simulink model "ssc_pneumatic_actuator"  (R2014a)
settings: Solver=ode23t  StartTime=0.0  StopTime=10  FixedStep=0.01  RelTol=1e-3
undefined symbols (not defined in the file): sigbuilder_block
libraries: fl_lib x50, nesl_utility x8
Description:
  | Pneumatic Actuation Circuit
  | 
  | This example shows how the Foundation Library pneumatic components
  | can be used to model a controlled pneumatic actuator. The Directional
  | 5-way valve, Double-acting pneumatic actuator and Pipe blocks
  | are masked subsystems created from Foundation Library blocks.
  | Double-click on the blocks to view the subsystem parameters. Select
  | the block and type ctrl-U to view its construction from fundamental
  | components. The pipe and actuator components include a simple
  | convection model of heat loss.
  | 
  | In the simulation, the directional valve is initially moved to its
  | maximum positive displacement, and the actuator moves the load
  | until it reaches the actuator end stop. The valve is then centered, and
  | the load is held. Next the valve moves to its maximum negative
  | displacement and the actuator retracts to its minimum length. The
  | valve is then centered again, locking the load in position.
  | 
  | 
  | Copyright 2008-2014 The MathWorks, Inc.
settings Model: Creator=MathWorks  LastModifiedBy=rodralez
settings DataIOCC: SignalLoggingSaveFormat=ModelDataLogs
settings OptimizationCC: ExpressionDepthLimit=2147483647
settings DebuggingCC: UnderspecifiedInitializationDetection=Classic  SolverPrmCheckMsg=none  FcnCallInpInsideContextMsg=UseLocalSettings  StateNameClashWarn=warning  StrictBusMsg=Warning
settings GRTTargetCC: CombineOutputUpdateFcns=off  GRTInterface=on

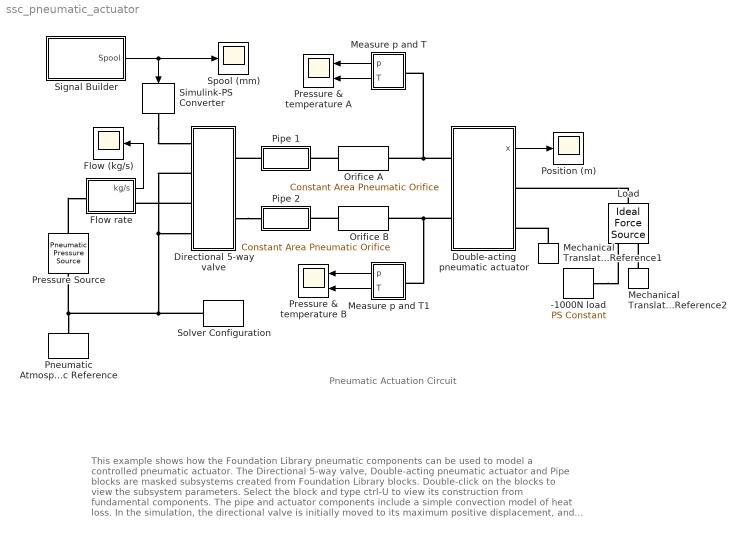
== system ssc_pneumatic_actuator ==
  note: Pneumatic Actuation Circuit
  note: This example shows how the Foundation Library pneumatic components can be used to model a controlled
      | pneumatic actuator. The Directional 5-way valve, Double-acting pneumatic actuator and Pipe blocks
      | are masked subsystems created from Foundation Library blocks. Double-click on the blocks to view
      | the subsystem parameters. Select the block and type ctrl-U to view its construction from fundamental
      | components. The pipe and actuator components include a simple convection model of heat loss.
      | In the simulation, the directional valve is initially moved to its maximum positive displacement,
      | and the actuator moves the load until it reaches the actuator end stop. The valve is then centered,
      | and the load is held. Next the valve moves to its maximum negative displacement and the actuator
      | retracts to its minimum length. The valve is then centered again, locking the load in position.
  -1000N load : fl_lib/Physical Signals/Sources/PS Constant  constant=-1000
  Directional 5-way valve : Subsystem  mask(Directional 5-way valve){Cd=0.82, x_max=5, A_max=5, x_lap=0.2, A_leak=0.0001}
      mask prompts: Cd "Discharge coefficient:"; x_max "Displacement limit (mm)"; A_max "Maximum orifice area (mm^2)"; x_lap "Displacement range for leakage (mm)"; A_leak "Leakage area at x=0 (mm^2)"
      mask help: Models a directional 5-way valve assuming a linear relationship between valve position and valve area. Input supply pressure should be applied to port P, and the actuator connected to ports A and B. Ports R and S are the return paths for ports A and B respectively.
      mask Display:
      | image(imread('valve_5_3.jpg'))
      | color('red')
      | port_label('Lconn',1,'x')
      | port_label('Lconn',2,'R')
      | port_label('Lconn',3,'P')
      | port_label('Lconn',4,'S')
      | port_label('Rconn',1,'A')
      | port_label('Rconn',2,'B')
  Double-acting pneumatic actuator : Subsystem  mask(Double-acting pneumatic actuator){A=0.002, L=0.2, V0=1e-4, mass=1, lambda=200, mass_total=3, c_act=870, k=100, Ta=293.15, x0=0, p0_A=101325, T_A=293.15, p0_B=101325, T_B=293.15, T_act=293.15}
      mask prompts: A "Cross-sectional area (m^2)"; L "Length of travel (m)"; V0 "Dead volume (m^3)"; mass "Piston mass (kg)"; lambda "Mechanical damping (N/m/s)"; mass_total "Actuator total mass (kg)"; c_act "Actuator material specific heat (J/kg/K)"; k "Convective heat transfer coefficient (W/(m^2*K)"; Ta "Ambient temperature (K)"; x0 "Initial length (m)"; p0_A "Chamber A initial pressure (Pa)"; T_A "Chamber A initial temperature (K)"; p0_B "Chamber B initial pressure (Pa)"; T_B "Chamber B initial temperature (K)"; T_act "Actuator initial temperature (K)"
      mask help: This block models a double-acting pneumatic actuator by using two Foundation Library Piston Chamber components connected in parallel.
      mask init:
      | D = sqrt(4*A/pi);
  Flow (kg/s) : Scope
      settings: TimeRange=10  YMin=-0.0005  YMax=0.002  SaveName=ScopeData2
  Flow rate : Subsystem
  Load : fl_lib/Mechanical/Mechanical Sources/Ideal Force Source
  Measure p and T : Subsystem
  Measure p and T1 : Subsystem
  Mechanical Translational Reference1 : fl_lib/Mechanical/Translational Elements/Mechanical Translational Reference
  Mechanical Translational Reference2 : fl_lib/Mechanical/Translational Elements/Mechanical Translational Reference
  Orifice A : fl_lib/Pneumatic/Pneumatic Elements/Constant Area Pneumatic Orifice  Cd=0.82  Area=1.5 mm^2  G_specify=off  G_priority=High  G=0 kg/s  Q1_specify=off  Q1_priority=High  Q1=0 J/s  Q2_specify=off  Q2_priority=High  Q2=0 J/s  p1_specify=off  p1_priority=High  p1=1e+5 Pa  p2_specify=off  p2_priority=High  p2=1e+5 Pa  T1_specify=off  T1_priority=High  T1=300 K  T2_specify=off  T2_priority=High  T2=300 K
  Orifice B : fl_lib/Pneumatic/Pneumatic Elements/Constant Area Pneumatic Orifice  Cd=0.82  Area=1.2 mm^2  G_specify=off  G_priority=High  G=0 kg/s  Q1_specify=off  Q1_priority=High  Q1=0 J/s  Q2_specify=off  Q2_priority=High  Q2=0 J/s  p1_specify=off  p1_priority=High  p1=1e+5 Pa  p2_specify=off  p2_priority=High  p2=1e+5 Pa  T1_specify=off  T1_priority=High  T1=300 K  T2_specify=off  T2_priority=High  T2=300 K
  Pipe 1 : Subsystem  mask(Pipe Volume){L=1, D=2.5e-3, t=1e-3, rho=1500, c_p=1250, k=100, Ta=293.15, p0=101325, T0=293.15}
      mask prompts: L "Pipe length (m)"; D "Internal diameter (m)"; t "Wall thickness (m)"; rho "Pipe wall density (kg/m^3)"; c_p "Pipe wall specific heat (J/kg/K)"; k "Convective heat transfer coefficient (W/(m^2*K)"; Ta "Ambient temperature"; p0 "Initial pressure (Pa)"; T0 "Initial temperature (K)"
      mask help: Simple model of a pneumatic pipe. Model comprises a constant volume of gas with convective heat transfer to the pipe wall and from the pipe wall to the environment.
  Pipe 2 : Subsystem  mask(Pipe Volume){L=1, D=2.5e-3, t=1e-3, rho=1500, c_p=1250, k=100, Ta=293.15, p0=101325, T0=293.15}
      mask prompts: L "Pipe length (m)"; D "Internal diameter (m)"; t "Wall thickness (m)"; rho "Pipe wall density (kg/m^3)"; c_p "Pipe wall specific heat (J/kg/K)"; k "Convective heat transfer coefficient (W/(m^2*K)"; Ta "Ambient temperature"; p0 "Initial pressure (Pa)"; T0 "Initial temperature (K)"
      mask help: Simple model of a pneumatic pipe. Model comprises a constant volume of gas with convective heat transfer to the pipe wall and from the pipe wall to the environment.
  Pneumatic Atmospheric Reference : fl_lib/Pneumatic/Pneumatic Elements/Pneumatic Atmospheric Reference
  Position (m) : Scope
      settings: TimeRange=10  YMin=-0.1  YMax=0.3  SaveName=ScopeData5
  Pressure Source : fl_lib/Pneumatic/Pneumatic Sources/Pneumatic Pressure Source  pressure_difference_reference=6 bar
  Pressure & temperature A : Scope  NumInputPorts=2
      settings: TimeRange=10  YMin=0~100  YMax=10~600  SaveName=ScopeData3
  Pressure & temperature B : Scope  NumInputPorts=2
      settings: TimeRange=10  YMin=0~200  YMax=8~600
  Signal Builder : Subsystem  Tag=STV Subsys  LoadFcn=sigbuilder_block('load');  StartFcn=sigbuilder_block('start');  StopFcn=sigbuilder_block('stop');  ClipboardFcn=sigbuilder_block('clipboard');  mask(Sigbuilder block){}
      mask help: Sigbuilder GUI
      mask init:
      | if ~strcmp(get_param(bdroot(gcbh),'SimulationStatus'),'stopped') tuvar = sigbuilder_block('maskInit'); end
      settings: CopyFcn=sigbuilder_block('copy');  DeleteFcn=sigbuilder_block('delete');  ModelCloseFcn=sigbuilder_block('modelClose');  PreSaveFcn=sigbuilder_block('preSave');  PauseFcn=sigbuilder_block('pause')  ContinueFcn=sigbuilder_block('continue')  NameChangeFcn=sigbuilder_block('namechange');  OpenFcn=sigbuilder_block('open',[124.873 467.793 550.402 399.593 ]);  CloseFcn=sigbuilder_block('close');
      mask Display: plot(0,0,100,100,[10,10,40,40,10],[80,20,20,80,80],[40,10],[50,50], [40,27,10],[65,72,56],[40,25,25,10],[28,28,43,43]);
  Simulink-PS Converter : nesl_utility/Simulink-PS Converter  PhysicalDomain=network_engine_domain  SubClassName=ps_input  LeftPortType=input  RightPortType=output  PseudoPeriodic=off  Frequencies=[]  NoiseDistribution=none  NoiseParameters=[]  Unit=mm  AffineConversion=off  InputFiltering=off  SimscapeFilterOrder=1  InputFilterTimeConstant=.001  UdotUserProvided=0
  Solver Configuration : nesl_utility/Solver Configuration  PhysicalDomain=network_engine_domain  SubClassName=solver  LeftPortType=input  RightPortType=generic  Accelerate=off  Tones=[]  Harmonics=[]  SimulateNoise=off  Profile=off  UseLocalSampling=off  EnableSwitchedLinearOptims=on  FrequencyDomain=off  UseCCode=off  RelTol=0.001  AbsTol=1e-06  MinStep=1e-09  ToWorkspace=off  DoDC=off  ResidualTolerance=1e-9  UseLocalSolver=off  LocalSolverChoice=NE_BACKWARD_EULER_ADVANCER  LocalSolverSampleTime=.001  DoFixedCost=off  MaxNonlinIter=3  MaxModeIter=2  LinearAlgebra=Sparse  DelaysMemoryBudget=1024  AutomaticFiltering=on  FilteringTimeConstant=0.001
  Spool (mm) : Scope
      settings: TimeRange=10  YMin=-6  YMax=6
  wires:
  Double-acting pneumatic actuator/1(x) -> Position (m)/1
  Flow rate/1(kg/s) -> Flow (kg/s)/1
  Measure p and T/1(p) -> Pressure & temperature A/1
  Measure p and T/2(T) -> Pressure & temperature A/2
  Signal Builder/1(Spool) -> Simulink-PS Converter/1, Spool (mm)/1
  Measure p and T1/1(p) -> Pressure & temperature B/1
  Measure p and T1/2(T) -> Pressure & temperature B/2
  connections:
  Directional 5-way valve/LConn2 -- Pressure Source/RConn1 -- Pneumatic Atmospheric Reference/LConn1 -- Solver Configuration/RConn1 -- Directional 5-way valve/LConn4
  Mechanical Translational Reference1/LConn1 -- Double-acting pneumatic actuator/RConn2
  Pressure Source/LConn1 -- Flow rate/LConn1
  Directional 5-way valve/LConn3 -- Flow rate/RConn1
  Directional 5-way valve/RConn2 -- Pipe 2/RConn1
  Simulink-PS Converter/RConn1 -- Directional 5-way valve/LConn1
  Pipe 1/LConn1 -- Directional 5-way valve/RConn1
  Double-acting pneumatic actuator/LConn2 -- Orifice B/LConn1 -- Measure p and T1/LConn1
  Double-acting pneumatic actuator/LConn1 -- Orifice A/RConn1 -- Measure p and T/LConn1
  Orifice A/LConn1 -- Pipe 1/RConn1
  Orifice B/RConn1 -- Pipe 2/LConn1
  Load/LConn1 -- Double-acting pneumatic actuator/RConn1
  Mechanical Translational Reference2/LConn1 -- Load/RConn2
  -1000N load/RConn1 -- Load/RConn1

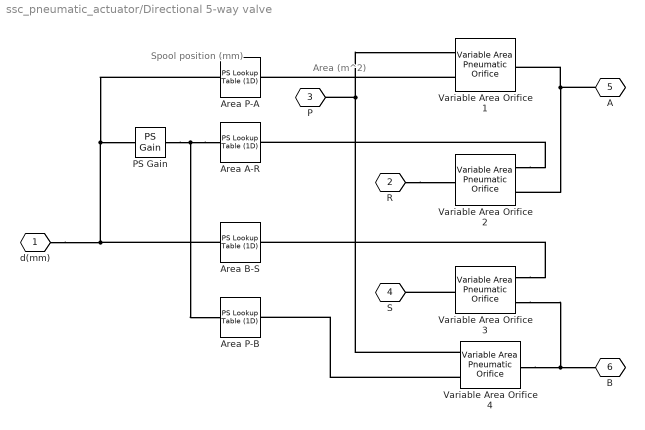
== system ssc_pneumatic_actuator/Directional 5-way valve ==
  note: Area (m^2)
  note: Spool position (mm)
  Area A-R : fl_lib/Physical Signals/Lookup Tables/PS Lookup Table (1D)  x_t=[-x_max -x_lap 0 x_lap x_max 2*x_max]  y_t=[0 0 A_leak 2*A_leak A_max A_max]*1e-6  interp_method=1  extrap_method=1
  Area B-S : fl_lib/Physical Signals/Lookup Tables/PS Lookup Table (1D)  x_t=[-x_max -x_lap 0 x_lap x_max 2*x_max]  y_t="[0 0  A_leak 2*A_leak A_max A_max]*1e-6"  interp_method=1  extrap_method=1
  Area P-A : fl_lib/Physical Signals/Lookup Tables/PS Lookup Table (1D)  x_t=[-x_max -x_lap 0 x_lap x_max 2*x_max]  y_t=[0 0 A_leak 2*A_leak A_max A_max]*1e-6  interp_method=1  extrap_method=1
  Area P-B : fl_lib/Physical Signals/Lookup Tables/PS Lookup Table (1D)  x_t=[-x_max -x_lap 0 x_lap x_max 2*x_max]  y_t=[0 0 A_leak 2*A_leak A_max A_max]*1e-6  interp_method=1  extrap_method=1
  PS Gain : fl_lib/Physical Signals/Functions/PS Gain  gain=-1
  Variable Area Orifice {1..4} (4 alike) : fl_lib/Pneumatic/Pneumatic Elements/Variable Area Pneumatic Orifice  Cd=Cd  Area0=1e-10 m^2  G_specify=off  G_priority=High  G=0 kg/s  Q1_specify=off  Q1_priority=High  Q1=0 J/s  Q2_specify=off  Q2_priority=High  Q2=0 J/s  p1_specify=off  p1_priority=High  p1=1e+5 Pa  p2_specify=off  p2_priority=High  p2=1e+5 Pa  T1_specify=off  T1_priority=High  T1=300 K  T2_specify=off  T2_priority=High  T2=300 K
  d(mm) : PMIOPort  Tag=PMCPort  Port=1  Side=Left
  R : PMIOPort  Tag=PMCPort  Port=2  Side=Left
  P : PMIOPort  Tag=PMCPort  Port=3  Side=Left
  S : PMIOPort  Tag=PMCPort  Port=4  Side=Left
  A : PMIOPort  Tag=PMCPort  Port=5  Side=Right
  B : PMIOPort  Tag=PMCPort  Port=6  Side=Right
  connections:
  Area B-S/LConn1 -- d(mm)/RConn1 -- PS Gain/LConn1 -- Area P-A/LConn1
  Variable Area Orifice 1/LConn2 -- Area P-A/RConn1
  Variable Area Orifice 4/LConn1 -- P/RConn1 -- Variable Area Orifice 1/LConn1
  Variable Area Orifice 2/LConn1 -- A/RConn1 -- Variable Area Orifice 1/RConn1
  R/RConn1 -- Variable Area Orifice 2/RConn1
  Variable Area Orifice 4/LConn2 -- Area P-B/RConn1
  Variable Area Orifice 3/LConn1 -- B/RConn1 -- Variable Area Orifice 4/RConn1
  Area A-R/LConn1 -- PS Gain/RConn1 -- Area P-B/LConn1
  Variable Area Orifice 2/LConn2 -- Area A-R/RConn1
  Variable Area Orifice 3/LConn2 -- Area B-S/RConn1
  Variable Area Orifice 3/RConn1 -- S/RConn1

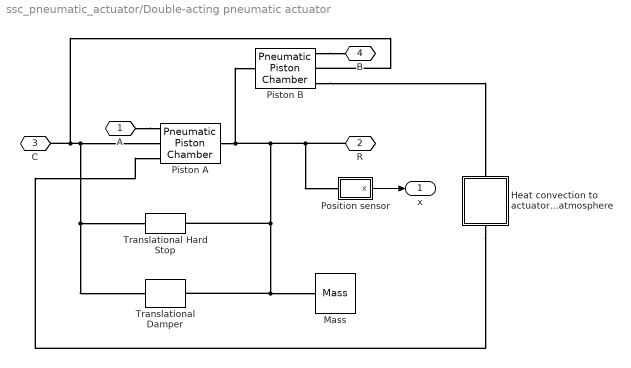
== system ssc_pneumatic_actuator/Double-acting pneumatic actuator ==
  Heat convection to actuator body and atmosphere : Subsystem
  Mass : fl_lib/Mechanical/Translational Elements/Mass  mass=mass kg  v_specify=on  v_priority=High  v=0 m/s  f_specify=off  f_priority=High  f=0 N
  Piston A : fl_lib/Pneumatic/Pneumatic Elements/Pneumatic Piston Chamber  Area=A m^2  x0=x0 m  V0=V0 m^3  or=1  gas_flow_specify=off  gas_flow_priority=High  gas_flow=0 kg/s  heat_flow_specify=off  heat_flow_priority=High  heat_flow=0 J/s  pressure_specify=on  pressure_priority=High  pressure=p0_A Pa  temperature_specify=on  temperature_priority=High  temperature=T_A K  heat_exch_flow_specify=off  heat_exch_flow_priority=High  heat_exch_flow=0 J/s  velocity_specify=off  velocity_priority=High  velocity=0 m/s  force_specify=off  force_priority=High  force=0 N
  Piston B : fl_lib/Pneumatic/Pneumatic Elements/Pneumatic Piston Chamber  Area=A m^2  x0=L-x0 m  V0=V0 m^3  or=2  gas_flow_specify=off  gas_flow_priority=High  gas_flow=0 kg/s  heat_flow_specify=off  heat_flow_priority=High  heat_flow=0 J/s  pressure_specify=on  pressure_priority=High  pressure=p0_B Pa  temperature_specify=on  temperature_priority=High  temperature=T_B K  heat_exch_flow_specify=off  heat_exch_flow_priority=High  heat_exch_flow=0 J/s  velocity_specify=off  velocity_priority=High  velocity=0 m/s  force_specify=off  force_priority=High  force=0 N
  Position sensor : Subsystem
  Translational Damper : fl_lib/Mechanical/Translational Elements/Translational Damper  D=lambda N/(m/s)  v_specify=off  v_priority=High  v=0 m/s  f_specify=off  f_priority=High  f=0 N
  Translational Hard Stop : fl_lib/Mechanical/Translational Elements/Translational Hard Stop  upper_bnd=L-x0 m  lower_bnd=-x0 m  stiff_up=1e+07 N/m  stiff_low=1e+07 N/m  D_up=1500 N/(m/s)  D_low=1500 N/(m/s)  v_specify=off  v_priority=High  v=0 m/s  f_specify=off  f_priority=High  f=0 N  x_specify=on  x_priority=High  x=0 m
  A : PMIOPort  Port=1  Side=Left
  R : PMIOPort  Port=2  Side=Right
  C : PMIOPort  Port=3  Side=Right
  B : PMIOPort  Port=4  Side=Left
  x : Outport
  wires:
  Position sensor/1(x) -> x/1
  connections:
  A/RConn1 -- Piston A/LConn1
  Piston B/LConn2 -- Translational Hard Stop/RConn1 -- Translational Damper/RConn1 -- Piston A/LConn2 -- C/RConn1
  Piston B/LConn1 -- B/RConn1
  R/RConn1 -- Piston A/RConn1 -- Piston B/RConn1 -- Translational Hard Stop/LConn1 -- Translational Damper/LConn1 -- Mass/LConn1 -- Position sensor/LConn1
  Piston B/LConn3 -- Heat convection to actuator body and atmosphere/LConn1
  Heat convection to actuator body and atmosphere/RConn1 -- Piston A/LConn3

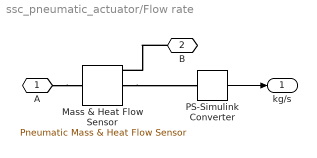
== system ssc_pneumatic_actuator/Flow rate ==
  Mass & Heat Flow Sensor : fl_lib/Pneumatic/Pneumatic Sensors/Pneumatic Mass & Heat Flow Sensor
  PS-Simulink Converter : nesl_utility/PS-Simulink Converter  PhysicalDomain=network_engine_domain  SubClassName=ps_output  LeftPortType=input  RightPortType=output  PseudoPeriodic=off  Frequencies=[]  Unit=kg/s  AffineConversion=off
  A : PMIOPort  Port=1  Side=Left
  B : PMIOPort  Port=2  Side=Right
  kg/s : Outport
  wires:
  PS-Simulink Converter/1 -> kg/s/1
  connections:
  Mass & Heat Flow Sensor/RConn2 -- PS-Simulink Converter/LConn1
  B/RConn1 -- Mass & Heat Flow Sensor/RConn1
  A/RConn1 -- Mass & Heat Flow Sensor/LConn1

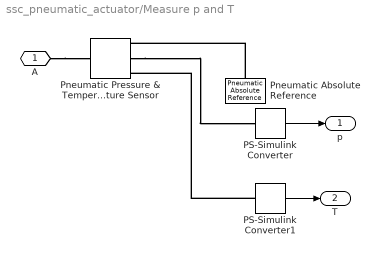
== system ssc_pneumatic_actuator/Measure p and T ==
  PS-Simulink Converter : nesl_utility/PS-Simulink Converter  PhysicalDomain=network_engine_domain  SubClassName=ps_output  LeftPortType=input  RightPortType=output  PseudoPeriodic=off  Frequencies=[]  Unit=bar  AffineConversion=off
  PS-Simulink Converter1 : nesl_utility/PS-Simulink Converter  PhysicalDomain=network_engine_domain  SubClassName=ps_output  LeftPortType=input  RightPortType=output  PseudoPeriodic=off  Frequencies=[]  Unit=K  AffineConversion=off
  Pneumatic Absolute Reference : fl_lib/Pneumatic/Pneumatic Elements/Pneumatic Absolute Reference
  Pneumatic Pressure & Temperature Sensor : fl_lib/Pneumatic/Pneumatic Sensors/Pneumatic Pressure & Temperature Sensor
  A : PMIOPort  Port=1  Side=Left
  p : Outport
  T : Outport  Port=2
  wires:
  PS-Simulink Converter1/1 -> T/1
  PS-Simulink Converter/1 -> p/1
  connections:
  PS-Simulink Converter1/LConn1 -- Pneumatic Pressure & Temperature Sensor/RConn3
  A/RConn1 -- Pneumatic Pressure & Temperature Sensor/LConn1
  Pneumatic Pressure & Temperature Sensor/RConn2 -- PS-Simulink Converter/LConn1
  Pneumatic Absolute Reference/LConn1 -- Pneumatic Pressure & Temperature Sensor/RConn1

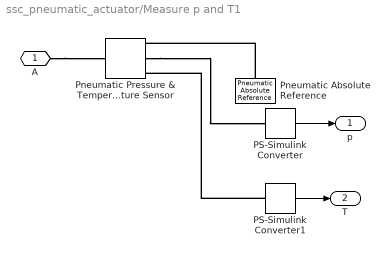
== system ssc_pneumatic_actuator/Measure p and T1 ==
  PS-Simulink Converter : nesl_utility/PS-Simulink Converter  PhysicalDomain=network_engine_domain  SubClassName=ps_output  LeftPortType=input  RightPortType=output  PseudoPeriodic=off  Frequencies=[]  Unit=bar  AffineConversion=off
  PS-Simulink Converter1 : nesl_utility/PS-Simulink Converter  PhysicalDomain=network_engine_domain  SubClassName=ps_output  LeftPortType=input  RightPortType=output  PseudoPeriodic=off  Frequencies=[]  Unit=K  AffineConversion=off
  Pneumatic Absolute Reference : fl_lib/Pneumatic/Pneumatic Elements/Pneumatic Absolute Reference
  Pneumatic Pressure & Temperature Sensor : fl_lib/Pneumatic/Pneumatic Sensors/Pneumatic Pressure & Temperature Sensor
  A : PMIOPort  Port=1  Side=Left
  p : Outport
  T : Outport  Port=2
  wires:
  PS-Simulink Converter/1 -> p/1
  PS-Simulink Converter1/1 -> T/1
  connections:
  Pneumatic Absolute Reference/LConn1 -- Pneumatic Pressure & Temperature Sensor/RConn1
  Pneumatic Pressure & Temperature Sensor/RConn2 -- PS-Simulink Converter/LConn1
  A/RConn1 -- Pneumatic Pressure & Temperature Sensor/LConn1
  PS-Simulink Converter1/LConn1 -- Pneumatic Pressure & Temperature Sensor/RConn3

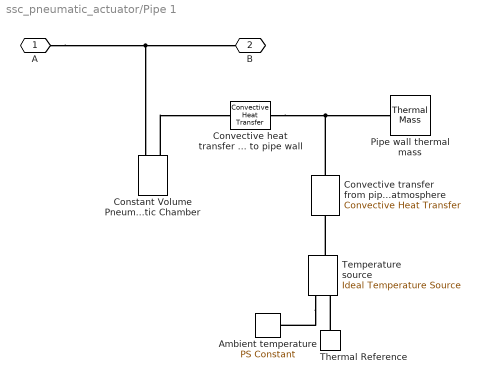
== system ssc_pneumatic_actuator/Pipe 1 ==
  Ambient temperature : fl_lib/Physical Signals/Sources/PS Constant  constant=Ta
  Constant Volume Pneumatic Chamber : fl_lib/Pneumatic/Pneumatic Elements/Constant Volume Pneumatic Chamber  Volume=L*pi*D^2/4 m^3  gas_flow_specify=off  gas_flow_priority=High  gas_flow=0 kg/s  heat_flow_specify=off  heat_flow_priority=High  heat_flow=0 J/s  pressure_specify=on  pressure_priority=High  pressure=p0 Pa  temperature_specify=on  temperature_priority=High  temperature=T0 K  heat_exch_flow_specify=off  heat_exch_flow_priority=High  heat_exch_flow=0 J/s
  Convective heat transfer from air in pipe to pipe wall : fl_lib/Thermal/Thermal Elements/Convective Heat Transfer  area=pi*D*L m^2  heat_tr_coeff=k W/(m^2 * K)  Q_specify=off  Q_priority=High  Q=0 J/s  T_specify=off  T_priority=High  T=0 K
  Convective transfer from pipe to atmosphere : fl_lib/Thermal/Thermal Elements/Convective Heat Transfer  area=pi*D*L m^2  heat_tr_coeff=k W/(m^2 * K)  Q_specify=off  Q_priority=High  Q=0 J/s  T_specify=off  T_priority=High  T=0 K
  Pipe wall thermal mass : fl_lib/Thermal/Thermal Elements/Thermal Mass  mass=rho*pi*D*t*L kg  sp_heat=c_p J/kg/K  Q_specify=off  Q_priority=High  Q=0 J/s  T_specify=on  T_priority=High  T=T0 K
  Temperature source : fl_lib/Thermal/Thermal Sources/Ideal Temperature Source
  Thermal Reference : fl_lib/Thermal/Thermal Elements/Thermal Reference
  A : PMIOPort  Port=1  Side=Left
  B : PMIOPort  Port=2  Side=Right
  connections:
  A/RConn1 -- Constant Volume Pneumatic Chamber/LConn1 -- B/RConn1
  Constant Volume Pneumatic Chamber/LConn2 -- Convective heat transfer from air in pipe to pipe wall/LConn1
  Thermal Reference/LConn1 -- Temperature source/RConn2
  Temperature source/LConn1 -- Convective transfer from pipe to atmosphere/LConn1
  Convective transfer from pipe to atmosphere/RConn1 -- Pipe wall thermal mass/LConn1 -- Convective heat transfer from air in pipe to pipe wall/RConn1
  Temperature source/RConn1 -- Ambient temperature/RConn1

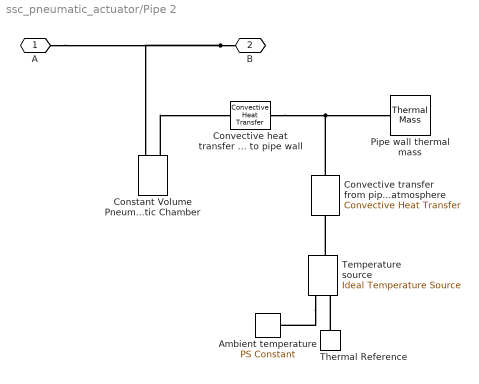
== system ssc_pneumatic_actuator/Pipe 2 ==
  Ambient temperature : fl_lib/Physical Signals/Sources/PS Constant  constant=Ta
  Constant Volume Pneumatic Chamber : fl_lib/Pneumatic/Pneumatic Elements/Constant Volume Pneumatic Chamber  Volume=L*pi*D^2/4 m^3  gas_flow_specify=off  gas_flow_priority=High  gas_flow=0 kg/s  heat_flow_specify=off  heat_flow_priority=High  heat_flow=0 J/s  pressure_specify=on  pressure_priority=High  pressure=p0 Pa  temperature_specify=on  temperature_priority=High  temperature=T0 K  heat_exch_flow_specify=off  heat_exch_flow_priority=High  heat_exch_flow=0 J/s
  Convective heat transfer from air in pipe to pipe wall : fl_lib/Thermal/Thermal Elements/Convective Heat Transfer  area=pi*D*L m^2  heat_tr_coeff=k W/(m^2 * K)  Q_specify=off  Q_priority=High  Q=0 J/s  T_specify=off  T_priority=High  T=0 K
  Convective transfer from pipe to atmosphere : fl_lib/Thermal/Thermal Elements/Convective Heat Transfer  area=pi*D*L m^2  heat_tr_coeff=k W/(m^2 * K)  Q_specify=off  Q_priority=High  Q=0 J/s  T_specify=off  T_priority=High  T=0 K
  Pipe wall thermal mass : fl_lib/Thermal/Thermal Elements/Thermal Mass  mass=rho*pi*D*t*L kg  sp_heat=c_p J/kg/K  Q_specify=off  Q_priority=High  Q=0 J/s  T_specify=on  T_priority=High  T=T0 K
  Temperature source : fl_lib/Thermal/Thermal Sources/Ideal Temperature Source
  Thermal Reference : fl_lib/Thermal/Thermal Elements/Thermal Reference
  A : PMIOPort  Port=1  Side=Left
  B : PMIOPort  Port=2  Side=Right
  connections:
  Temperature source/LConn1 -- Convective transfer from pipe to atmosphere/LConn1
  Temperature source/RConn1 -- Ambient temperature/RConn1
  Thermal Reference/LConn1 -- Temperature source/RConn2
  Convective transfer from pipe to atmosphere/RConn1 -- Pipe wall thermal mass/LConn1 -- Convective heat transfer from air in pipe to pipe wall/RConn1
  Constant Volume Pneumatic Chamber/LConn2 -- Convective heat transfer from air in pipe to pipe wall/LConn1
  B/RConn1 -- Constant Volume Pneumatic Chamber/LConn1 -- A/RConn1

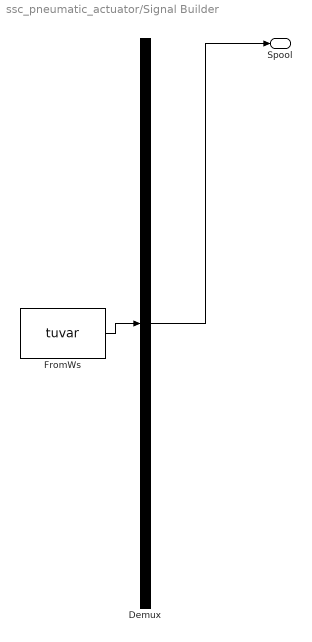
== system ssc_pneumatic_actuator/Signal Builder ==
  Demux : Demux  Tag=STV Demux  Outputs=1
  FromWs : FromWorkspace  Tag=STV FromWs  VariableName=tuvar  SampleTime=0
      SigBuilderData=|
      | common.afterFinalStr = 'Extrapolate'
      | common.sampleTime = 0
      | dataSet.timeRange = [0 10]
      | dataSet.name = 'Group 1'
      | sbobj.Groups.Name = 'Group 1'
      | sbobj.Groups.Signals.Name = 'Spool'
      | sbobj.Groups.Signals.XData = [0 0.98 1.22 3.54 3.66 4.86 4.98 7.62 7.84 10]
      | sbobj.Groups.Signals.YData = [0 0 5 5 -0.02 0 -5 -5 0 0]
  Spool : Outport  Tag=STV Outport
  wires:
  Demux/1 -> Spool/1
  FromWs/1 -> Demux/1

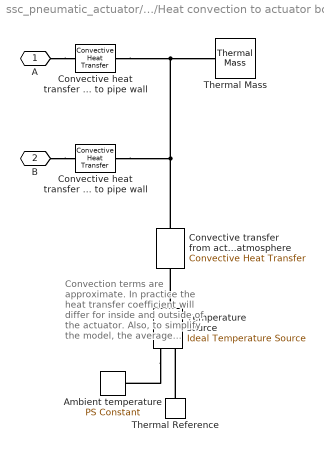
== system ssc_pneumatic_actuator/Double-acting pneumatic actuator/Heat convection to actuator body and atmosphere ==
  note: Convection terms are
      | approximate. In practice
      | the heat transfer coefficient
      | will differ for inside and
      | outside of the actuator.
      | Also, to simplify the model,
      | the average chamber area
      | is used.
  Ambient temperature : fl_lib/Physical Signals/Sources/PS Constant  constant=Ta
  Convective heat transfer from air in chamber A to pipe wall : fl_lib/Thermal/Thermal Elements/Convective Heat Transfer  area=2*A+pi*D*L/2 m^2  heat_tr_coeff=k W/(m^2 * K)  Q_specify=off  Q_priority=High  Q=0 J/s  T_specify=off  T_priority=High  T=0 K
  Convective heat transfer from air in chamber B to pipe wall : fl_lib/Thermal/Thermal Elements/Convective Heat Transfer  area=2*A+pi*D*L/2 m^2  heat_tr_coeff=k W/(m^2 * K)  Q_specify=off  Q_priority=High  Q=0 J/s  T_specify=off  T_priority=High  T=0 K
  Convective transfer from actuator to atmosphere : fl_lib/Thermal/Thermal Elements/Convective Heat Transfer  area=2*A+pi*D*L m^2  heat_tr_coeff=k W/(m^2 * K)  Q_specify=off  Q_priority=High  Q=0 J/s  T_specify=off  T_priority=High  T=0 K
  Temperature source : fl_lib/Thermal/Thermal Sources/Ideal Temperature Source
  Thermal Mass : fl_lib/Thermal/Thermal Elements/Thermal Mass  mass=mass_total kg  sp_heat=c_act J/kg/K  Q_specify=off  Q_priority=High  Q=0 J/s  T_specify=on  T_priority=High  T=T_act K
  Thermal Reference : fl_lib/Thermal/Thermal Elements/Thermal Reference
  A : PMIOPort  Port=1  Side=Left
  B : PMIOPort  Port=2  Side=Right
  connections:
  A/RConn1 -- Convective heat transfer from air in chamber A to pipe wall/LConn1
  Thermal Reference/LConn1 -- Temperature source/RConn2
  Temperature source/LConn1 -- Convective transfer from actuator to atmosphere/LConn1
  Convective transfer from actuator to atmosphere/RConn1 -- Convective heat transfer from air in chamber A to pipe wall/RConn1 -- Thermal Mass/LConn1 -- Convective heat transfer from air in chamber B to pipe wall/RConn1
  Temperature source/RConn1 -- Ambient temperature/RConn1
  B/RConn1 -- Convective heat transfer from air in chamber B to pipe wall/LConn1

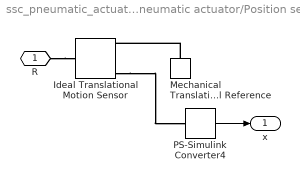
== system ssc_pneumatic_actuator/Double-acting pneumatic actuator/Position sensor ==
  Ideal Translational Motion Sensor : fl_lib/Mechanical/Mechanical Sensors/Ideal Translational Motion Sensor  offset=x0 m
  Mechanical Translational Reference : fl_lib/Mechanical/Translational Elements/Mechanical Translational Reference
  PS-Simulink Converter4 : nesl_utility/PS-Simulink Converter  PhysicalDomain=network_engine_domain  SubClassName=ps_output  LeftPortType=input  RightPortType=output  PseudoPeriodic=off  Frequencies=[]  Unit=m  AffineConversion=off
  R : PMIOPort  Port=1  Side=Left
  x : Outport
  wires:
  PS-Simulink Converter4/1 -> x/1
  connections:
  R/RConn1 -- Ideal Translational Motion Sensor/LConn1
  Ideal Translational Motion Sensor/RConn3 -- PS-Simulink Converter4/LConn1
  Mechanical Translational Reference/LConn1 -- Ideal Translational Motion Sensor/RConn1
